simulink library "commseqgen2"  (Simulink 6.0)
settings: Solver=ode45  SolverMode=SingleTasking  StartTime=0.0  StopTime=10.0  RelTol=1e-3
libraries: simulink x4, dspsrcs4 x4, commseqgen2 x2
settings Model: Creator=mikem  LastModifiedBy=akansal
settings DataIOCC: SignalLoggingName=logsOut
settings OptimizationCC: BooleanDataType=off
settings DebuggingCC: CheckExecutionContextPreStartOutputMsg=on  CheckExecutionContextRuntimeOutputMsg=on  SolverPrmCheckMsg=none
settings HardwareCC: TargetUnknown=on
settings SFSimCC: SFSimApplyToAllLibs=on  SFSimBuildMode=Incremental

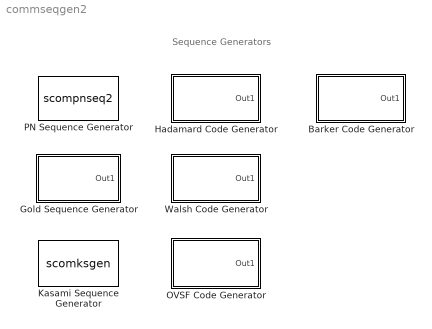
== system commseqgen2 ==
  note: Sequence Generators
  Barker Code Generator : Subsystem  PropExecContextAcrossSSBoundary=on  mask(Barker Code Generator){length=7, ts=1, frameBased=off, sampPerFrame=1}
      mask prompts: length "Code length:"; ts "Sample time:"; frameBased "Frame-based outputs"; sampPerFrame "Samples per frame:"
      mask help:
      | Generate a Barker Code of the specified length.
      |
      | The output code is in a bi-polar format with a {0, 1} to {1, -1} element mapping.
      mask init:
      | [bCode, sampPerFrame, eStr] = commblkbcgen(gcb,'init');
      | if (eStr.ecode == 1)
      | 	error(eStr.emsg);
      | end
      mask Help: helpview(commbhelp);
      mask StyleString: popup(1|2|3|4|5|7|11|13),edit,checkbox,edit
      mask CallbackString: ||commblkbcgen(gcb,'cbFrameBased');|
      mask Display: disp('Barker Code\nGenerator');
  Gold Sequence Generator : Subsystem  PropExecContextAcrossSSBoundary=on  mask(Gold Sequence Generator){genPoly1=[1 0 0 0 0 1 1], iniState1=[0 0 0 0 0 1], genPoly2=[1 1 0 0 1 1 1], iniState2=[0 0 0 0 0 1], index=0, shift=0, ts=1, frameBased=off, sampPerFrame=1, reset=off}
      mask prompts: genPoly1 "Preferred polynomial (1):"; iniState1 "Initial states (1):"; genPoly2 "Preferred polynomial (2):"; iniState2 "Initial states (2):"; index "Sequence index:"; ts "Sample time:"; frameBased "Frame-based outputs"; sampPerFrame "Samples per frame:"; reset "Reset on nonzero input"
      mask help:
      | Generate a Gold sequence from a set of sequences by specifying a preferred pair of polynomials.
      |
      | The polynomial parameter values represent the shift register connections. Enter these values as either a binary vector or a descending ordered polynomial to indicate the connection points.
      |
      | The initial states parameters are binary vectors that represent the starting state of the shift registers.
      |
      | The sequence index parameter denotes the single sequence outputted from the set of Gold sequences. Specify it as a scalar integer in the range [-2, 2^n-2] where n is the degree of the generator polynomial. The index values -2 and -1 correspond to the first and second PN sequences as generated by the preferred polynomials (1) and (2), respectively.
      |
      | The shift parameter is a scalar integer that produces an offset in the sequence.
      mask init:
      | [genPoly1, iniState1, genPoly2, iniState2, index, shift, rstPortLbl, eStr] = commblkgcgen(gcb, 'init');
      | if (eStr.ecode == 1)
      | 	error(eStr.emsg);
      | end
      mask Help: helpview(commbhelp);
      mask CallbackString: |||||||commblkgcgen(gcb,'cbFrameBased');||commblkgcgen(gcb,'cbReset');
      mask Display:
      | disp('Gold Sequence\nGenerator');
      | text(rstPortLbl.x, rstPortLbl.y, rstPortLbl.str);
  Hadamard Code Generator : Subsystem  PropExecContextAcrossSSBoundary=on  mask(Hadamard Code Generator){length=64, index=60, ts=1, frameBased=off, sampPerFrame=1}
      mask prompts: length "Code length:"; index "Code index:"; ts "Sample time:"; frameBased "Frame-based outputs"; sampPerFrame "Samples per frame:"
      mask help:
      | Generate a Hadamard Code from an orthogonal set of codes.
      |
      | The code index parameter is an integer scalar in the range [0, N-1] where N is the code length.  When incremented by 1, it corresponds to the row index of a Hadamard matrix of size N x N. N must be an integer power of 2.
      |
      | The output code is in a bipolar format with a {0, 1} to {1, -1} element mapping.
      mask init:
      | [hCode, sampPerFrame, eStr] = commblkhcgen(gcb,'init');
      | if (eStr.ecode == 1)
      | 	error(eStr.emsg);
      | end
      mask Help: helpview(commbhelp);
      mask CallbackString: |||commblkwcgen(gcb,'cbFrameBased');|
      mask Display: disp('Hadamard\nCode Generator');
  Kasami Sequence Generator : S-Function  FunctionName=scomksgen  Parameters=genPoly, iniState, codeIdx, shift, ts, frameBased, sampPerFrame, reset  mask(Kasami Sequence Generator){genPoly=[1 0 0 0 0 1 1], iniState=[0 0 0 0 0 1], codeIdx=0, shift=0, ts=1, frameBased=off, sampPerFrame=1, reset=off}
      mask prompts: genPoly "Generator polynomial:"; iniState "Initial states:"; codeIdx "Sequence index(es):"; ts "Sample time:"; frameBased "Frame-based outputs"; sampPerFrame "Samples per frame:"; reset "Reset on nonzero input"
      mask help:
      | Generate a Kasami sequence from the set of Kasami sequences by specifying the generator polynomial.
      |
      | The generator polynomial parameter value represents the shift register connections. Enter these values as either a binary vector or a descending ordered polynomial to indicate the connection points.
      |
      | The initial states parameter is a binary vector that represents the starting state of the shift register.
      |
      | The sequence index parameter denotes the single sequence outputted from the set of Kasami sequences. Specify it as a 2-element integer vector for the Large set of sequences or as a scalar integer for the Small set of sequences.
      |
      | The shift parameter is a scalar integer that produces an offset in the sequence.
      mask init:
      | [genPoly, codeIdx, shift, rstPortLbl, eStr] = commblkksgen(gcb, 'init');
      |  if (eStr.ecode == 1)
      | 	error(eStr.emsg);
      | end
      mask Help: helpview(commbhelp);
      mask CallbackString: |||||commblkksgen(gcb,'cbFrameBased');||
      mask Display:
      | disp('Kasami\nSequence\nGenerator');
      | text(rstPortLbl.x, rstPortLbl.y, rstPortLbl.str);
  OVSF Code Generator : Subsystem  PropExecContextAcrossSSBoundary=on  mask(OVSF Code Generator){spreadFact=64, index=60, ts=1, frameBased=off, sampPerFrame=1}
      mask prompts: spreadFact "Spreading factor:"; index "Code index:"; ts "Sample time:"; frameBased "Frame-based outputs"; sampPerFrame "Samples per frame:"
      mask help:
      | Generate an Orthogonal Variable Spreading Factor (OVSF) Code from a set of orthogonal codes.
      |
      | The code index parameter is an integer scalar in the range [0, N-1] where N is the spreading factor.  It corresponds to the bit-flipped row index of a Hadamard matrix of size N x N, when that is incremented by 1. N must be an integer power of 2.
      |
      | The output code is in a bipolar format with a {0,1} to {1, -1} element mapping.
      mask init:
      | [ovsfCode, sampPerFrame, eStr] = commblkovsfcgen(gcb,'init');
      | if (eStr.ecode == 1)
      | 	error(eStr.emsg);
      | end
      mask Help: helpview(commbhelp);
      mask CallbackString: |||commblkovsfcgen(gcb,'cbFrameBased');|
      mask Display: disp('OVSF Code\nGenerator');
  PN Sequence Generator : S-Function  FunctionName=scompnseq2  Parameters=poly, ini_sta, shift, Ts, frameBased, sampPerFrame, reset  mask(PN Sequence Generator){poly=[1 0 0 0 0 1 1], ini_sta=[0 0 0 0 0 1], shift=0, Ts=1, frameBased=off, sampPerFrame=1, reset=off}
      mask prompts: poly "Generator polynomial:"; ini_sta "Initial states:"; shift "Shift (or mask):"; Ts "Sample time:"; frameBased "Frame-based outputs"; sampPerFrame "Samples per frame:"; reset "Reset on nonzero input"
      mask help:
      | Generate a pseudonoise (PN) sequence using a linear feedback shift register whose configuration is specified by the Generator polynomial parameter.
      |
      | The generator polynomial parameter values represent the shift register connections. Enter these values as either a binary vector or a descending ordered polynomial to indicate the connection points.
      |
      | For the binary vector representation the first and last elements of the vector must be 1. For the descending ordered polynomial representation the last element of the vector must be 0.
      |
      | The initial states parameter is a binary vector that represents the starting state of the shift register.
      |
      | The shift parameter is a scalar integer that produces an offset in the PN sequence. As a result, the block outputs the sequence from a future instant in time. Alternatively, one can specify the mask parameter as a binary vector corresponding to the same shift.
      mask init:
      | [poly, shift, rstPortLbl, eStr] = commblkpnseq2(gcb,'init');
      | if eStr.ecode
      | 	error(eStr.emsg);
      | end
      mask Help: helpview(commbhelp);
      mask CallbackString: ||||commblkpnseq2(gcb,'cbFrameBased');||
      mask Display:
      | disp('PN Sequence\nGenerator');
      | text(rstPortLbl.x, rstPortLbl.y, rstPortLbl.str);
  Walsh Code Generator : Subsystem  PropExecContextAcrossSSBoundary=on  mask(Walsh Code Generator){length=64, index=60, ts=1, frameBased=off, sampPerFrame=1}
      mask prompts: length "Code length:"; index "Code index:"; ts "Sample time:"; frameBased "Frame-based outputs"; sampPerFrame "Samples per frame:"
      mask help:
      | Generate a Walsh Code from an orthogonal set of codes.
      |
      | The code index parameter is a scalar in the range [0, N-1] where N is the code length.  It corresponds to the number of zero crossings in an output code of length N. N must be an integer power of 2.
      |
      | The output code is in a bipolar format with a {0, 1} to {1, -1} element mapping.
      mask init:
      | [wCode, sampPerFrame, eStr] = commblkwcgen(gcb,'init');
      | if (eStr.ecode == 1)
      | 	error(eStr.emsg);
      | end
      mask Help: helpview(commbhelp);
      mask CallbackString: |||commblkwcgen(gcb,'cbFrameBased');|
      mask Display: disp('Walsh Code\nGenerator');

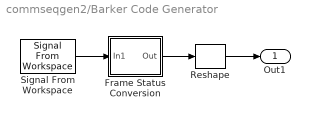
== system commseqgen2/Barker Code Generator ==
  Frame Status Conversion : Subsystem  AncestorBlock=dspsigattribs/Frame Status Conversion  PropExecContextAcrossSSBoundary=on  mask(Frame Status Conversion){growRefPort=off, outframe=Sample-based}
      mask prompts: growRefPort "Inherit output frame status from Ref input port"; outframe "Output signal:"
      mask help: Specify the frame status of the output signal.
      mask init:
      | [p, str] = dspblkfrmconv('init');
      mask Help: web(dspbhelp);
      mask StyleString: checkbox,popup(Frame-based|Sample-based)
      mask CallbackString: dspblkfrmconv|
      mask Display:
      | port_label(p.in1,   p.i1,  p.i1s);
      | port_label(p.in2,   p.i2,  p.i2s);
      | port_label(p.out, p.o1, p.o1s);
      | disp(str)
  Reshape : simulink/Math Operations/Reshape  OutputDimensionality=1-D array  OutputDimensions=[1,1]
  Signal From Workspace : dspsrcs4/Signal From Workspace  X=bCode  Ts=ts  nsamps=sampPerFrame  OutputAfterFinalValue=Cyclic repetition
  Out1 : Outport
  wires:
  Frame Status Conversion/1(Out) -> Reshape/1
  Signal From Workspace/1 -> Frame Status Conversion/1(In1)
  Reshape/1 -> Out1/1

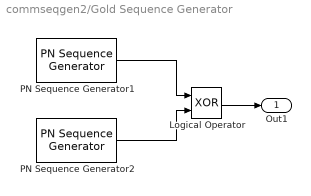
== system commseqgen2/Gold Sequence Generator ==
  Logical Operator : Logic  Operator=XOR  AllPortsSameDT=off  OutDataTypeMode=Specify via dialog  LogicDataType=float('double')
  PN Sequence Generator1 : commseqgen2/PN Sequence Generator  poly=genPoly1  ini_sta=iniState1  shift=shift  Ts=ts  frameBased=off  sampPerFrame=sampPerFrame  reset=off
  PN Sequence Generator2 : commseqgen2/PN Sequence Generator  poly=genPoly2  ini_sta=iniState2  shift=shift + index  Ts=ts  frameBased=off  sampPerFrame=sampPerFrame  reset=off
  Out1 : Outport
  wires:
  PN Sequence Generator1/1 -> Logical Operator/1
  PN Sequence Generator2/1 -> Logical Operator/2
  Logical Operator/1 -> Out1/1

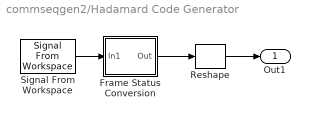
== system commseqgen2/Hadamard Code Generator ==
  Frame Status Conversion : Subsystem  AncestorBlock=dspsigattribs/Frame Status Conversion  PropExecContextAcrossSSBoundary=on  mask(Frame Status Conversion){growRefPort=off, outframe=Sample-based}
      mask prompts: growRefPort "Inherit output frame status from Ref input port"; outframe "Output signal:"
      mask help: Specify the frame status of the output signal.
      mask init:
      | [p, str] = dspblkfrmconv('init');
      mask Help: web(dspbhelp);
      mask StyleString: checkbox,popup(Frame-based|Sample-based)
      mask CallbackString: dspblkfrmconv|
      mask Display:
      | port_label(p.in1,   p.i1,  p.i1s);
      | port_label(p.in2,   p.i2,  p.i2s);
      | port_label(p.out, p.o1, p.o1s);
      | disp(str)
  Reshape : simulink/Math Operations/Reshape  OutputDimensionality=1-D array  OutputDimensions=[1,1]
  Signal From Workspace : dspsrcs4/Signal From Workspace  X=hCode  Ts=ts  nsamps=sampPerFrame  OutputAfterFinalValue=Cyclic repetition
  Out1 : Outport
  wires:
  Frame Status Conversion/1(Out) -> Reshape/1
  Signal From Workspace/1 -> Frame Status Conversion/1(In1)
  Reshape/1 -> Out1/1

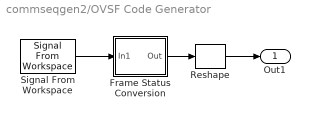
== system commseqgen2/OVSF Code Generator ==
  Frame Status Conversion : Subsystem  AncestorBlock=dspsigattribs/Frame Status Conversion  PropExecContextAcrossSSBoundary=on  mask(Frame Status Conversion){growRefPort=off, outframe=Sample-based}
      mask prompts: growRefPort "Inherit output frame status from Ref input port"; outframe "Output signal:"
      mask help: Specify the frame status of the output signal.
      mask init:
      | [p, str] = dspblkfrmconv('init');
      mask Help: web(dspbhelp);
      mask StyleString: checkbox,popup(Frame-based|Sample-based)
      mask CallbackString: dspblkfrmconv|
      mask Display:
      | port_label(p.in1,   p.i1,  p.i1s);
      | port_label(p.in2,   p.i2,  p.i2s);
      | port_label(p.out, p.o1, p.o1s);
      | disp(str)
  Reshape : simulink/Math Operations/Reshape  OutputDimensionality=1-D array  OutputDimensions=[1,1]
  Signal From Workspace : dspsrcs4/Signal From Workspace  X=ovsfCode  Ts=ts  nsamps=sampPerFrame  OutputAfterFinalValue=Cyclic repetition
  Out1 : Outport
  wires:
  Signal From Workspace/1 -> Frame Status Conversion/1(In1)
  Frame Status Conversion/1(Out) -> Reshape/1
  Reshape/1 -> Out1/1

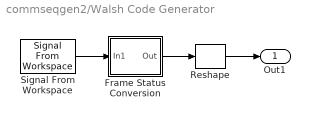
== system commseqgen2/Walsh Code Generator ==
  Frame Status Conversion : Subsystem  AncestorBlock=dspsigattribs/Frame Status Conversion  PropExecContextAcrossSSBoundary=on  mask(Frame Status Conversion){growRefPort=off, outframe=Sample-based}
      mask prompts: growRefPort "Inherit output frame status from Ref input port"; outframe "Output signal:"
      mask help: Specify the frame status of the output signal.
      mask init:
      | [p, str] = dspblkfrmconv('init');
      mask Help: web(dspbhelp);
      mask StyleString: checkbox,popup(Frame-based|Sample-based)
      mask CallbackString: dspblkfrmconv|
      mask Display:
      | port_label(p.in1,   p.i1,  p.i1s);
      | port_label(p.in2,   p.i2,  p.i2s);
      | port_label(p.out, p.o1, p.o1s);
      | disp(str)
  Reshape : simulink/Math Operations/Reshape  OutputDimensionality=1-D array  OutputDimensions=[1,1]
  Signal From Workspace : dspsrcs4/Signal From Workspace  X=wCode  Ts=ts  nsamps=sampPerFrame  OutputAfterFinalValue=Cyclic repetition
  Out1 : Outport
  wires:
  Signal From Workspace/1 -> Frame Status Conversion/1(In1)
  Frame Status Conversion/1(Out) -> Reshape/1
  Reshape/1 -> Out1/1

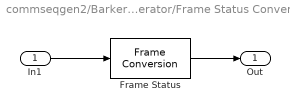
== system commseqgen2/Barker Code Generator/Frame Status Conversion ==
  In1 : Inport  LatchInput=off
  Frame Status : FrameConversion  OutFrame=Sample based
  Out : Outport
  wires:
  In1/1 -> Frame Status/1
  Frame Status/1 -> Out/1

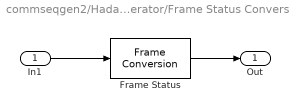
== system commseqgen2/Hadamard Code Generator/Frame Status Conversion ==
  In1 : Inport  LatchInput=off
  Frame Status : FrameConversion  OutFrame=Sample based
  Out : Outport
  wires:
  In1/1 -> Frame Status/1
  Frame Status/1 -> Out/1

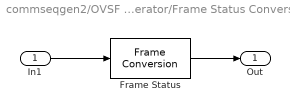
== system commseqgen2/OVSF Code Generator/Frame Status Conversion ==
  In1 : Inport  LatchInput=off
  Frame Status : FrameConversion  OutFrame=Sample based
  Out : Outport
  wires:
  Frame Status/1 -> Out/1
  In1/1 -> Frame Status/1

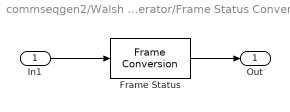
== system commseqgen2/Walsh Code Generator/Frame Status Conversion ==
  In1 : Inport  LatchInput=off
  Frame Status : FrameConversion  OutFrame=Sample based
  Out : Outport
  wires:
  Frame Status/1 -> Out/1
  In1/1 -> Frame Status/1
